simulink library "INT_ACCtl_Demand"  (R2016b)
settings: Solver=VariableStepAuto  StartTime=0.0  StopTime=10.0  RelTol=1e-3
settings Model: Creator=Administrator  LastModifiedBy=Administrator

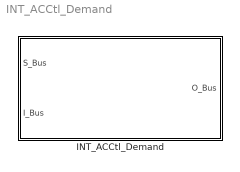
== system INT_ACCtl_Demand ==
  INT_ACCtl_Demand : Subsystem

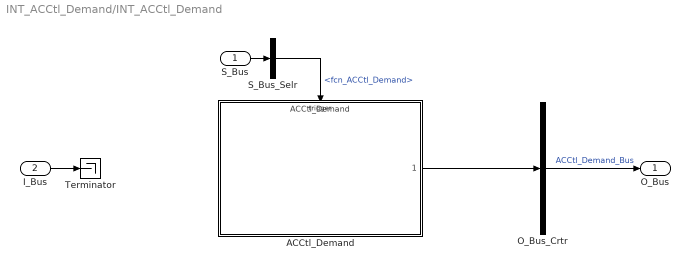
== system INT_ACCtl_Demand/INT_ACCtl_Demand ==
  S_Bus : Inport
  I_Bus : Inport  Port=2
  ACCtl_Demand : ModelReference  ModelNameDialog=ACCtl_Demand  SimulationMode=Normal  ModelReferenceVersion=1.2  TriggerPortName=function  TriggerPortTriggerType=function-call  TriggerPortStatesWhenEnabling=held
  O_Bus_Crtr : BusCreator  Inputs=1
  S_Bus_Selr : BusSelector  OutputSignals=fcn_ACCtl_Demand
  Terminator : Terminator
  O_Bus : Outport
  wires:
  S_Bus_Selr/1 -> ACCtl_Demand/Trigger  "<fcn_ACCtl_Demand>"
  S_Bus/1 -> S_Bus_Selr/1
  I_Bus/1 -> Terminator/1
  O_Bus_Crtr/1 -> O_Bus/1  "ACCtl_Demand_Bus"
  ACCtl_Demand/1 -> O_Bus_Crtr/1
